simulink model "titled3"  (R2015b)
settings: Solver=VariableStepAuto  StartTime=0.0  StopTime=10  RelTol=1e-3
libraries: dspmathops x2, dsparch4 x1
settings Model: Creator=Lukas  LastModifiedBy=Lukas

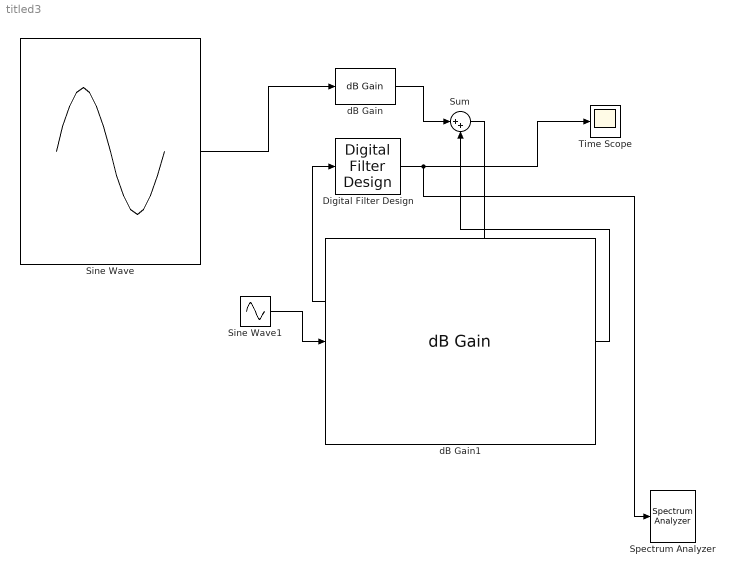
== system titled3 ==
  Digital Filter Design : dsparch4/Digital Filter Design  mwdsp_browser_bugfix_var=off
  Sine Wave : Sin  Frequency=100  SampleTime=1/8000
  Sine Wave1 : Sin  Frequency=500  SampleTime=1/8000
  Spectrum Analyzer : SpectrumAnalyzer
  Sum : Sum  Inputs=|++
  Time Scope : Scope
  dB Gain : dspmathops/dB Gain  dB=0  intype=Amplitude
  dB Gain1 : dspmathops/dB Gain  dB=0  intype=Amplitude
  wires:
  Sine Wave1/1 -> dB Gain1/1
  Sine Wave/1 -> dB Gain/1
  dB Gain/1 -> Sum/1
  dB Gain1/1 -> Sum/2
  Sum/1 -> Digital Filter Design/1
  Digital Filter Design/1 -> Spectrum Analyzer/1, Time Scope/1
